simulink model "voltage-control-of-inverter"  (R2023a)
settings: Solver=ode45  StartTime=0.0  StopTime=0.1  MaxStep=1e-7  MinStep=1e-8  RelTol=1e-3
libraries: spsMosfetLib x4, spsSeriesRLCBranchLib x4, spsRMSLib x3, spsVoltageMeasurementLib x3, spsCurrentMeasurementLib x2, eePwmGenerator x2, slpidlib x1, spsDCVoltageSourceLib x1, sps_lib x1
settings Model: Creator=AbdulfattahMolade  LastModifiedBy=mkoda
settings SolverCC: ZeroCrossAlgorithm=Adaptive

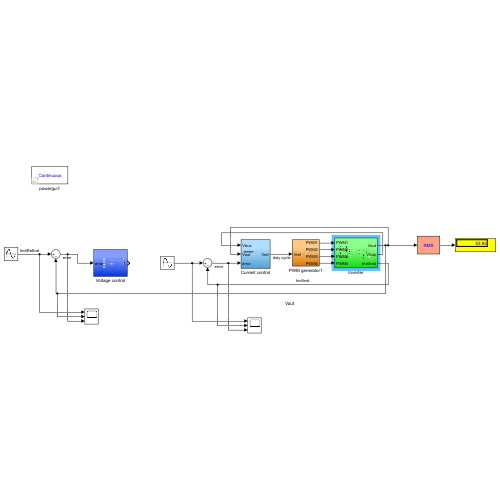
[thumbnail: Simulink's stored preview of the top-level diagram]
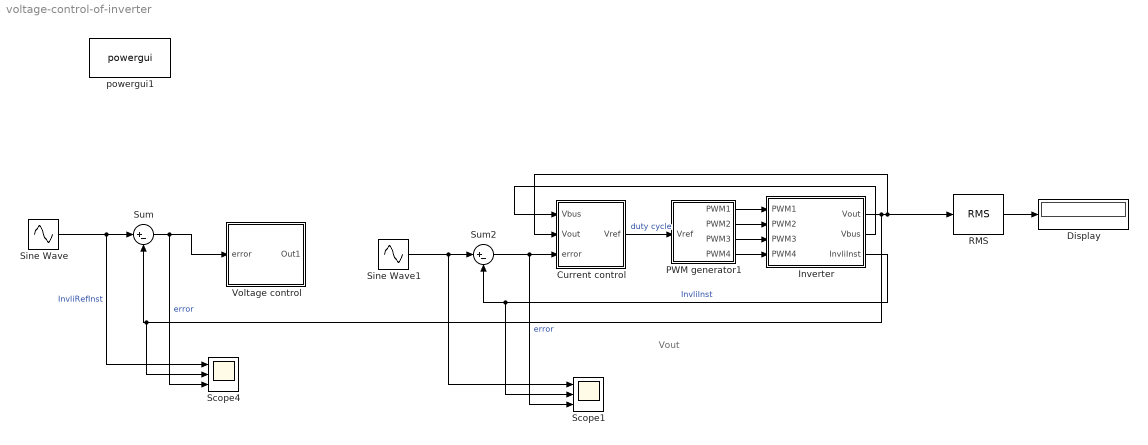
== system voltage-control-of-inverter ==
  note: Vout
  Current control : Subsystem
  Display : Display
  Inverter : Subsystem
  PWM generator1 : Subsystem
  RMS : spsRMSLib/RMS  TrueRMS=on  Freq=50  RMSInit=0  Ts=0
  Scope1 : Scope  NumInputPorts=3
  Scope4 : Scope  NumInputPorts=3
  Sine Wave : Sin  Amplitude=325.4  Frequency=2*pi*50  SampleTime=0
  Sine Wave1 : Sin  Frequency=2*pi*50  SampleTime=0
  Sum : Sum  Inputs=|+-
  Sum2 : Sum  Inputs=|+-
  Voltage control : Subsystem
  powergui1 : sps_lib/powergui  Priority=1  SimulationMode=Continuous  SampleTime=50e-6  frequency=60  Iterations=50  frequencyindice=0  Pbase=100e6  ErrMax=1e-4  UnitsV=kV  UnitsW=MW  buscounter=0  FunctionMessages=off  echomessages=off  EnableUseOfTLC=off  CurrentSourceSwitches=off  DisableSnubberDevices=off  DisableRonSwitches=off  DisableVfSwitches=off  DisplayEquations=off  AutomaticDiscreteSolvers=off  SolverType=Tustin/Backward Euler (TBE)  Interpol=off  ExternalGateDelay=off  methode=off  Ts=100  x0status=blocks  SPID=on  SwTol=0  HookPort=off  NonlinearTolerance=1e-4  nMaxIteration=100  ContinueOnMaxIteration=off  RestoreLinks=warning  ResistiveCurrentMeasurement=off  Frange=[0:2:500]  Ylog=off  Xlog=on  ShowGrid=off  save=off  variable=ZData  structure=0  ZoomFFT=off  StartTime=0.0  cycles=1  DisplayStyle=1  fundamental=60  FreqAxis=off  MaxFrequency=1000  frequencyindicesteady=1  RmsSteady=1  display=off
  wires:
  Sine Wave/1 -> Scope4/1, Sum/1  "InvliRefInst"
  Inverter/1(Vout) -> Current control/2(Vout), RMS/1, Scope4/2, Sum/2
  Inverter/3(InvliInst) -> Sum2/2, Scope1/2  "InvliInst"
  Sum2/1 -> Scope1/3, Current control/3(error)  "error"
  Inverter/2(Vbus) -> Current control/1(Vbus)
  Sum/1 -> Scope4/3, Voltage control/1(error)  "error"
  RMS/1 -> Display/1
  Current control/1(Vref) -> PWM generator1/1(Vref)  "duty cycle"
  PWM generator1/1(PWM1) -> Inverter/1(PWM1)
  PWM generator1/2(PWM2) -> Inverter/2(PWM2)
  PWM generator1/3(PWM3) -> Inverter/3(PWM3)
  PWM generator1/4(PWM4) -> Inverter/4(PWM4)
  Sine Wave1/1 -> Scope1/1, Sum2/1

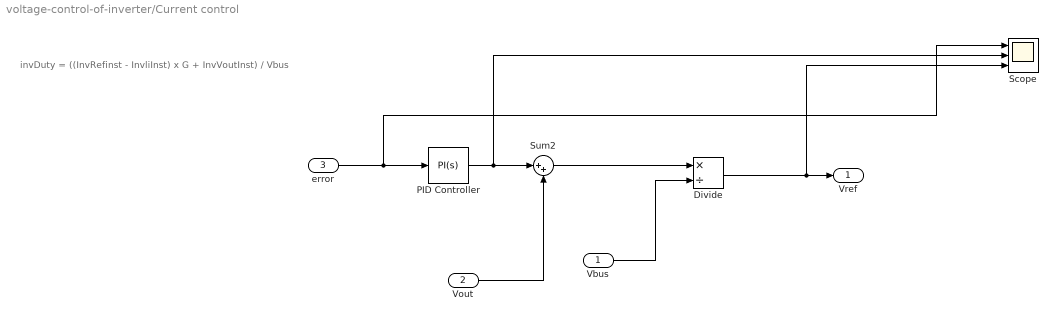
== system voltage-control-of-inverter/Current control ==
  note: invDuty = ((InvRefinst - InvliInst) x G + InvVoutInst) / Vbus
  Vbus : Inport
  Vout : Inport  Port=2
  error : Inport  Tag=error  Port=3
  Divide : Product  Inputs=*/
  PID Controller : slpidlib/PID Controller  Controller=PI  Form=Parallel  TimeDomain=Continuous-time  UseExternalTs=off  SampleTime=-1  IntegratorMethod=Forward Euler  FilterMethod=Forward Euler  ControllerParametersSource=internal  P=203.75796  I=32.48408  UseKiTs=off  D=0  N=100  UseFilter=on  TunerSelectOption=Transfer Function Based (PID Tuner App)  InitialConditionSource=internal  InitialConditionForIntegrator=0  InitialConditionForFilter=0  DifferentiatorICPrevScaledInput=0  ExternalReset=none  TrackingMode=off  Kt=1  LimitOutput=off  SatLimitsSource=internal  UpperSaturationLimit=inf  LowerSaturationLimit=-inf  LinearizeAsGain=on  AntiWindupMode=none  Kb=1  LimitIntegrator=off  UpperIntegratorSaturationLimit=inf  LowerIntegratorSaturationLimit=-inf  POutMin=[]  POutMax=[]  IOutMin=[]  IOutMax=[]  DOutMin=[]  DOutMax=[]  NOutMin=[]  NOutMax=[]  SumOutMin=[]  SumOutMax=[]  SaturationOutMin=[]  SaturationOutMax=[]  PParamMin=[]  PParamMax=[]  IParamMin=[]  IParamMax=[]  DParamMin=[]  DParamMax=[]  NParamMin=[]  NParamMax=[]  KbParamMin=[]  KbParamMax=[]  KtParamMin=[]  KtParamMax=[]  KbOutMin=[]  KbOutMax=[]  KtOutMin=[]  KtOutMax=[]  IntegratorOutMin=[]  IntegratorOutMax=[]  FilterOutMin=[]  FilterOutMax=[]  SumI1OutMin=[]  SumI1OutMax=[]  SumI2OutMin=[]  SumI2OutMax=[]  SumI3OutMin=[]  SumI3OutMax=[]  SumI4OutMin=[]  SumI4OutMax=[]  SumDOutMin=[]  SumDOutMax=[]  DifferentiatorOutMin=[]  DifferentiatorOutMax=[]  FilterDiffOutCoefMin=[]  FilterDiffOutCoefMax=[]  ReciprocalOutMin=[]  ReciprocalOutMax=[]  SumDenOutMin=[]  SumDenOutMax=[]  SumNumOutMin=[]  SumNumOutMax=[]  DivideOutMin=[]  DivideOutMax=[]  UdiffTsProdOutMin=[]  UdiffTsProdOutMax=[]  NTsProdOutMin=[]  NTsProdOutMax=[]  UintegralTsProdOutMin=[]  UintegralTsProdOutMax=[]  UngainTsProdOutMin=[]  UngainTsProdOutMax=[]  ClampingZeroOutDataTypeStr=Inherit: Inherit via back propagation  ClampingZeroOutMin=[]  ClampingZeroOutMax=[]  FilterDenConstantOutDataTypeStr=Inherit: Inherit via back propagation  FilterDenConstantOutMin=[]  FilterDenConstantOutMax=[]  PCopyOutDataTypeStr=Inherit: Inherit via back propagation  PCopyOutMin=[]  PCopyOutMax=[]  NCopyOutDataTypeStr=Inherit: Inherit via back propagation  NCopyOutMin=[]  NCopyOutMax=[]  IntegratorContinuousStateAttributes=''  IntegratorStateMustResolveToSignalObject=off  IntegratorRTWStateStorageClass=Auto  FilterContinuousStateAttributes=''  FilterStateMustResolveToSignalObject=off  FilterRTWStateStorageClass=Auto  ParallelPVariant=InternalParameters  IdealPVariant=Disabled  IVariant=InternalParameters  DVariant=Disabled  IntegratorVariant=Continuous  SatVariant=Disabled  AWVariant=Passthrough  PCopyVariant=Disabled  TRVariant=Disabled  FdbkBlocksVariant=Forward  IdealPFdbkVariant=Disabled  SatFdbkVariant=Disabled  DerivativeFilterVariant=Disabled  NVariant=Disabled  NCopyVariant=Disabled_SignalSpec  FilterICVariant=Disabled  IntegratorICVariant=InternalICs  ExternalResetVariant=Disabled  TRSumVariant=Passthrough  SumFdbkVariant=Disabled  SumVariant=Sum_PI  TsampFilterVariant=InternalTs  TsampNgainVariant=Passthrough  TsampIntegralVariant=Disabled_SignalSpec  ExternalSaturationOutDataTypeStr=Inherit: Same as second input
  Scope : Scope  NumInputPorts=3
  Sum2 : Sum  Inputs=|++
  Vref : Outport
  wires:
  Sum2/1 -> Divide/1
  Vout/1 -> Sum2/2
  PID Controller/1 -> Scope/2, Sum2/1
  error/1 -> Scope/1, PID Controller/1
  Vbus/1 -> Divide/2
  Divide/1 -> Scope/3, Vref/1

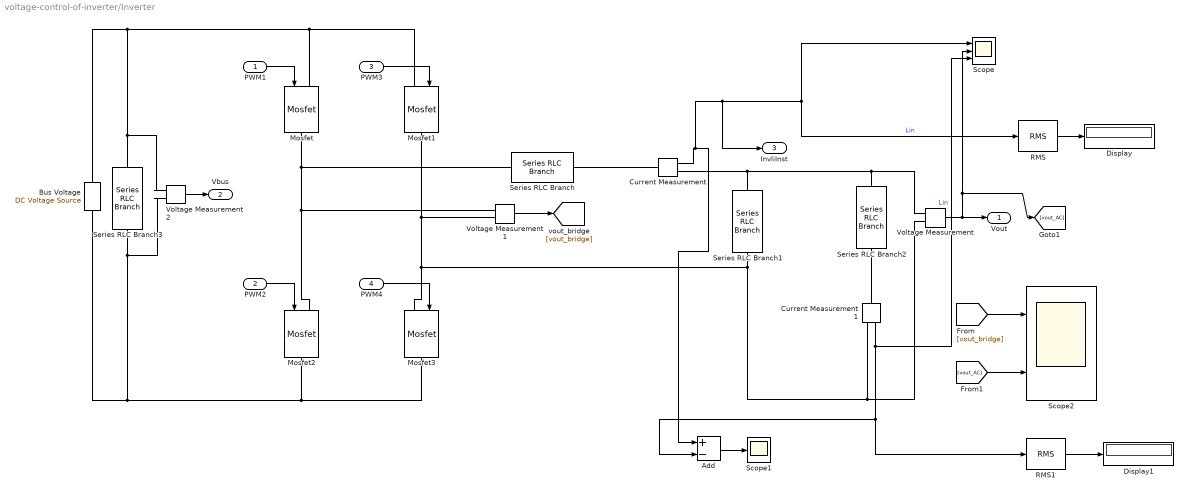
== system voltage-control-of-inverter/Inverter ==
  PWM1 : Inport
  PWM2 : Inport  Port=2
  PWM3 : Inport  Port=3
  PWM4 : Inport  Port=4
  Add : Sum  Inputs=+-
  Bus Voltage : spsDCVoltageSourceLib/DC Voltage Source  Amplitude=400  Measurements=None
  Current Measurement : spsCurrentMeasurementLib/Current Measurement  PhasorSimulation=off  OutputType=Complex  PSBequivalent=0
  Current Measurement1 : spsCurrentMeasurementLib/Current Measurement  PhasorSimulation=off  OutputType=Complex  PSBequivalent=0
  Display : Display
  Display1 : Display
  Mosfet{,1..3} (4 alike) : spsMosfetLib/Mosfet  Ron=0.1  Lon=0  Rd=0.01  Vfd=0  IC=0  Rs=1e5  Cs=inf  Measurements=off
  RMS : spsRMSLib/RMS  TrueRMS=on  Freq=50  RMSInit=0  Ts=0
  RMS1 : spsRMSLib/RMS  TrueRMS=on  Freq=50  RMSInit=0  Ts=0
  Scope : Scope  NumInputPorts=3
  Scope1 : Scope
  Scope2 : Scope  NumInputPorts=2
  Series RLC Branch : spsSeriesRLCBranchLib/Series RLC Branch  LConnTagsString=__new0  RConnTagsString=__new0  BranchType=RL  Resistance=0.001  Inductance=3.3e-3  SetiL0=off  InitialCurrent=0  Capacitance=1e-6  Setx0=off  InitialVoltage=0  Measurements=None
  Series RLC Branch1 : spsSeriesRLCBranchLib/Series RLC Branch  LConnTagsString=__new0  RConnTagsString=__new0  BranchType=RC  Resistance=0.0042  Inductance=3.3e-3  SetiL0=off  InitialCurrent=0  Capacitance=22e-6  Setx0=off  InitialVoltage=0  Measurements=Branch voltage
  Series RLC Branch2 : spsSeriesRLCBranchLib/Series RLC Branch  LConnTagsString=__new0  RConnTagsString=__new0  BranchType=R  Resistance=100  Inductance=1e-3  SetiL0=off  InitialCurrent=0  Capacitance=1e-6  Setx0=off  InitialVoltage=0  Measurements=None
  Series RLC Branch3 : spsSeriesRLCBranchLib/Series RLC Branch  LConnTagsString=__new0  RConnTagsString=__new0  BranchType=RC  Resistance=0.0042  Inductance=3.3e-3  SetiL0=off  InitialCurrent=0  Capacitance=500e-6  Setx0=off  InitialVoltage=0  Measurements=Branch voltage
  Voltage Measurement : spsVoltageMeasurementLib/Voltage Measurement  PhasorSimulation=off  OutputType=Complex  PSBequivalent=0
  Voltage Measurement1 : spsVoltageMeasurementLib/Voltage Measurement  PhasorSimulation=off  OutputType=Complex  PSBequivalent=0
  Voltage Measurement2 : spsVoltageMeasurementLib/Voltage Measurement  PhasorSimulation=off  OutputType=Complex  PSBequivalent=0
  Vout : Outport
  Vbus : Outport  Port=2
  InvliInst : Outport  Port=3
  wires:
  Voltage Measurement2/1 -> Vbus/1
  PWM1/1 -> Mosfet/1
  PWM2/1 -> Mosfet2/1
  Current Measurement/1 -> InvliInst/1, RMS/1, Scope/1, Add/1  "Lin"
  PWM4/1 -> Mosfet3/1
  PWM3/1 -> Mosfet1/1
  Voltage Measurement/1 -> Scope/2, [vout_AC], Vout/1
  Voltage Measurement1/1 -> [vout_bridge]
  [vout_bridge] -> Scope2/1
  [vout_AC] -> Scope2/2
  RMS/1 -> Display/1
  RMS1/1 -> Display1/1
  Current Measurement1/1 -> Scope/3, RMS1/1, Add/2  "Lin"
  Add/1 -> Scope1/1
  connections:
  Current Measurement/LConn1 -- Series RLC Branch/RConn1
  Mosfet1/RConn1 -- Voltage Measurement1/LConn2 -- Mosfet3/LConn1 -- Current Measurement1/RConn1 -- Voltage Measurement/LConn2 -- Series RLC Branch1/RConn1
  Mosfet/RConn1 -- Series RLC Branch/LConn1 -- Voltage Measurement1/LConn1 -- Mosfet2/LConn1
  Bus Voltage/RConn1 -- Voltage Measurement2/LConn1 -- Series RLC Branch3/LConn1 -- Mosfet1/LConn1 -- Mosfet/LConn1
  Bus Voltage/LConn1 -- Voltage Measurement2/LConn2 -- Series RLC Branch3/RConn1 -- Mosfet2/RConn1 -- Mosfet3/RConn1
  Series RLC Branch1/LConn1 -- Voltage Measurement/LConn1 -- Series RLC Branch2/LConn1 -- Current Measurement/RConn1
  Series RLC Branch2/RConn1 -- Current Measurement1/LConn1

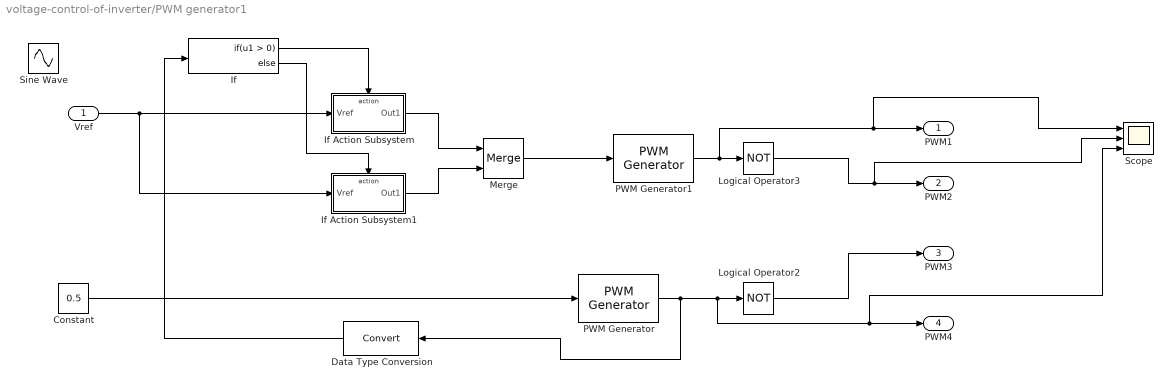
== system voltage-control-of-inverter/PWM generator1 ==
  Vref : Inport
  Constant : Constant  Value=0.5
  Data Type Conversion : DataTypeConversion  SaturateOnIntegerOverflow=off  RndMeth=Floor
  If : If
  If Action Subsystem : Subsystem  TreatAsAtomicUnit=on
  If Action Subsystem1 : Subsystem  TreatAsAtomicUnit=on
  Logical Operator2 : Logic  Operator=NOT  AllPortsSameDT=off  OutDataTypeStr=boolean
  Logical Operator3 : Logic  Operator=NOT  AllPortsSameDT=off  OutDataTypeStr=boolean
  Merge : Merge
  PWM Generator : eePwmGenerator/PWM Generator  CarrCount=Up  Tper=1/50  Tdelay=0  Ts=0
  PWM Generator1 : eePwmGenerator/PWM Generator  CarrCount=Up  Tper=1/20000  Tdelay=0  Ts=0
  Scope : Scope  NumInputPorts=3
  Sine Wave : Sin  Frequency=2*pi*50  SampleTime=0
  PWM1 : Outport
  PWM2 : Outport  Port=2
  PWM3 : Outport  Port=3
  PWM4 : Outport  Port=4
  wires:
  Constant/1 -> PWM Generator/1
  If Action Subsystem/1(Out1) -> Merge/1
  If Action Subsystem1/1(Out1) -> Merge/2
  Logical Operator3/1 -> Scope/2, PWM2/1
  Logical Operator2/1 -> PWM3/1
  PWM Generator1/1 -> Scope/1, PWM1/1, Logical Operator3/1
  PWM Generator/1 -> Data Type Conversion/1, Scope/3, PWM4/1, Logical Operator2/1
  If/1 -> If Action Subsystem/Action
  If/2 -> If Action Subsystem1/Action
  Merge/1 -> PWM Generator1/1
  Vref/1 -> If Action Subsystem1/1(Vref), If Action Subsystem/1(Vref)
  Data Type Conversion/1 -> If/1

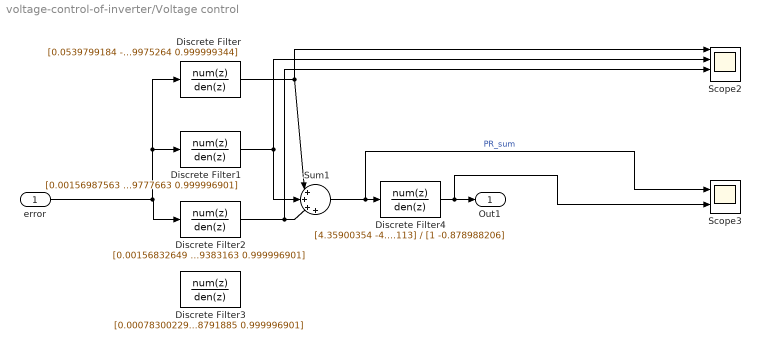
== system voltage-control-of-inverter/Voltage control ==
  error : Inport
  Discrete Filter : DiscreteFilter  Numerator=[0.0539799184 -0.10669072 0.0527239628]  Denominator=[1 -1.99975264 0.999999344]  SampleTime=1/20000
  Discrete Filter1 : DiscreteFilter  Numerator=[0.00156987563 0 -0.00156987563]  Denominator=[1 -1.99777663 0.999996901]  SampleTime=1/20000
  Discrete Filter2 : DiscreteFilter  Numerator=[0.00156832649 0 -0.00156832649]  Denominator=[1 -1.99383163 0.999996901]  SampleTime=1/20000
  Discrete Filter3 : DiscreteFilter  Numerator=[0.000783002295 0 -0.000783002295]  Denominator=[1 -1.98791885 0.999996901]  SampleTime=1/20000
  Discrete Filter4 : DiscreteFilter  Numerator=[4.35900354 -4.23082113]  Denominator=[1 -0.878988206]  SampleTime=1/20000
  Scope2 : Scope  NumInputPorts=4
  Scope3 : Scope  NumInputPorts=2
  Sum1 : Sum  Inputs=|++++
  Out1 : Outport
  wires:
  error/1 -> Discrete Filter/1, Discrete Filter1/1, Discrete Filter2/1
  Discrete Filter/1 -> Sum1/1, Scope2/1
  Discrete Filter2/1 -> Scope2/3, Sum1/3
  Sum1/1 -> Scope3/1, Discrete Filter4/1  "PR_sum"
  Discrete Filter1/1 -> Sum1/2, Scope2/2
  Discrete Filter4/1 -> Scope3/2, Out1/1

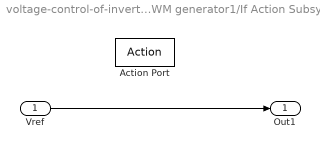
== system voltage-control-of-inverter/PWM generator1/If Action Subsystem ==
  Vref : Inport
  Action Port : ActionPort  ActionPortLabel=if(u1 > 0)
  Out1 : Outport
  wires:
  Vref/1 -> Out1/1

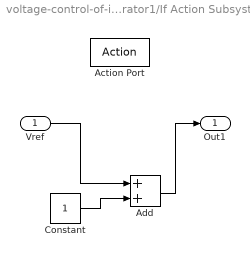
== system voltage-control-of-inverter/PWM generator1/If Action Subsystem1 ==
  Vref : Inport
  Action Port : ActionPort  ActionPortLabel=else
  Add : Sum
  Constant : Constant
  Out1 : Outport
  wires:
  Vref/1 -> Add/1
  Constant/1 -> Add/2
  Add/1 -> Out1/1
